simulink model "Model_SD_CIFB_k1"  (Simulink 10.0)
settings: Solver=VariableStepDiscrete  StartTime=0.0  StopTime=Tstop  RelTol=1e-3  EnableMultiTasking=on
values from neighbouring files (symbols this model uses):
  Amp = 10^(Av/20)*FS    (= 0.501187233627)    [run_Model_SD_CIFB_k2.m]
  fs = 2*BA*OSR    (= 2560000)    [run_Model_SD_CIFB_k2.m]
  OSR = 64    [run_Model_SD_CIFB_k2.m]
  ts = 1/fs    (= 3.90625e-07)    [run_Model_SD_CIFB_k2.m]
  win = 2*pi*fin    [run_Model_SD_CIFB_k2.m]
settings Model: LogicAnalyzerSignalOrdering=74cbdc39-9da7-4374-92c4-8284831780da  Creator=cellierr  LastModifiedBy=corentin.pichat
settings DataIOCC: LimitDataPoints=on
settings OptimizationCC: ExpressionDepthLimit=2147483647  InitFltsAndDblsToZero=on
settings DebuggingCC: SaveWithParameterizedLinksMsg=none  SolverPrmCheckMsg=warning  FcnCallInpInsideContextMsg=warning  StateNameClashWarn=warning
settings GRTTargetCC: TargetFcnLib=ansi_tfl_tmw.mat  GeneratePreprocessorConditionals=Disable all
settings ConfigComp: CovExternalEMLEnable=off  CovSFcnEnable=off

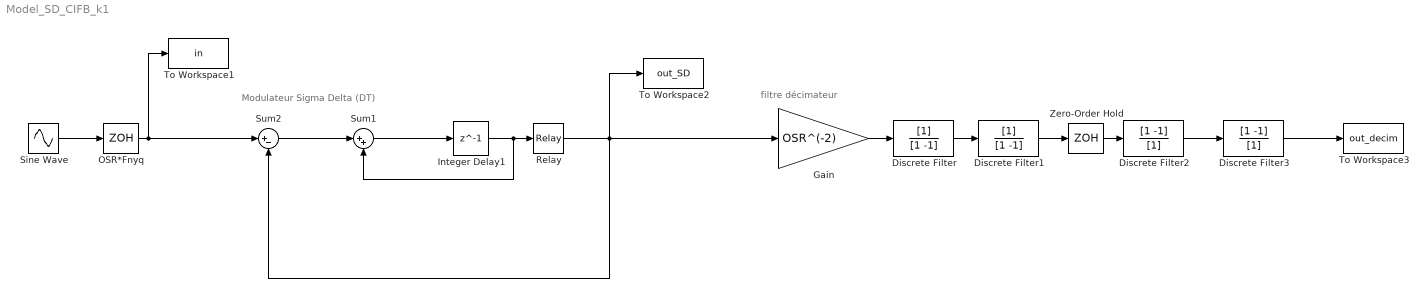
== system Model_SD_CIFB_k1 ==
  note: filtre décimateur
  note: Modulateur Sigma Delta (DT)
  Discrete Filter : DiscreteFilter  Denominator=[1 -1]
  Discrete Filter1 : DiscreteFilter  Denominator=[1 -1]
  Discrete Filter2 : DiscreteFilter  Numerator=[1 -1]  Denominator=[1]  SampleTime=ts*OSR
  Discrete Filter3 : DiscreteFilter  Numerator=[1 -1]  Denominator=[1]  SampleTime=ts*OSR
  Gain : Gain  Gain=OSR^(-2)  SaturateOnIntegerOverflow=on  OutDataTypeStr=Inherit: Same as input  ParamDataTypeStr=Inherit: Same as input
  Integer Delay1 : Delay  DelayLength=1
  OSR*Fnyq : ZeroOrderHold  SampleTime=1/(fs)
  Relay : Relay  OnSwitchValue=0  OffSwitchValue=0  OffOutputValue=-1
  Sine Wave : Sin  Amplitude=Amp  Frequency=win  SampleTime=0
  Sum1 : Sum  Inputs=|++
  Sum2 : Sum  Inputs=|+-
  To Workspace1 : ToWorkspace  VariableName=in  SampleTime=-1
  To Workspace2 : ToWorkspace  VariableName=out_SD  SampleTime=-1
  To Workspace3 : ToWorkspace  VariableName=out_decim  SampleTime=ts
  Zero-Order Hold : ZeroOrderHold  SampleTime=ts*OSR
  wires:
  Sine Wave/1 -> OSR*Fnyq/1
  Discrete Filter3/1 -> To Workspace3/1
  Sum1/1 -> Integer Delay1/1
  Sum2/1 -> Sum1/1
  OSR*Fnyq/1 -> To Workspace1/1, Sum2/1
  Integer Delay1/1 -> Relay/1, Sum1/2
  Gain/1 -> Discrete Filter/1
  Relay/1 -> Sum2/2, Gain/1, To Workspace2/1
  Discrete Filter1/1 -> Zero-Order Hold/1
  Discrete Filter/1 -> Discrete Filter1/1
  Zero-Order Hold/1 -> Discrete Filter2/1
  Discrete Filter2/1 -> Discrete Filter3/1
